simulink model "Drone"  (R2026a)
settings: Solver=VariableStepAuto  StopTime=50
values from neighbouring files (symbols this model uses):
  b = 3.13*10^(-5)    (= 3.13e-05)    [Drone_parameters.m]
  d = 7.5*10^(-7)    (= 7.5e-07)    [Drone_parameters.m]
  g = 9.81    [Drone_parameters.m]
  Ir = 6.5*10^(-5)    (= 6.5e-05)    [Drone_parameters.m]
  Ix = 7.5*10^(-3)    (= 0.0075)    [Drone_parameters.m]
  Iy = 7.5*10^(-3)    (= 0.0075)    [Drone_parameters.m]
  Iz = 1.3*10^(-2)    (= 0.013)    [Drone_parameters.m]
  kx = 0.01    [Drone_parameters.m]
  l = 0.23    [Drone_parameters.m]
  m = 0.65    [Drone_parameters.m]
libraries: slpidlib x6
settings Model: Creator=azmeh  LastModifiedBy=azmeh

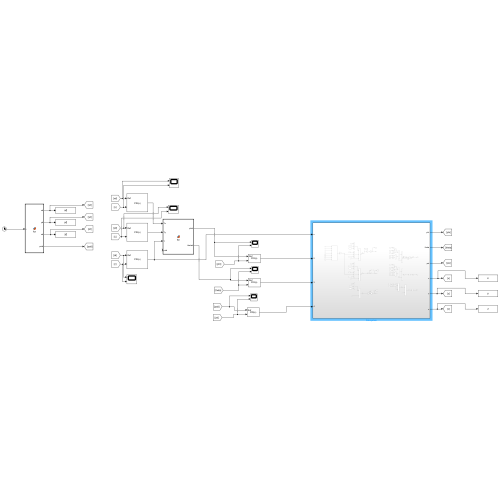
[thumbnail: Simulink's stored preview of the top-level diagram]
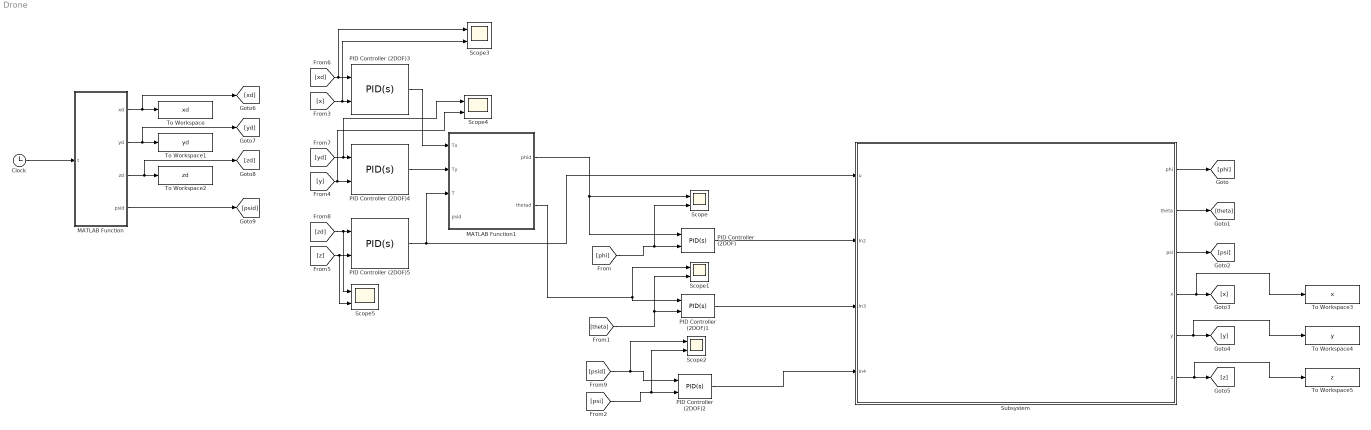
== system Drone ==
  Clock : Clock
  MATLAB Function : MATLAB Function  TreatAsAtomicUnit=on
  MATLAB Function1 : MATLAB Function  TreatAsAtomicUnit=on
  PID Controller (2DOF){,1..5} (6 alike) : slpidlib/PID Controller (2DOF)  Controller=PID  Form=Parallel  TimeDomain=Continuous-time  UseExternalTs=off  SampleTime=-1  IntegratorMethod=Forward Euler  FilterMethod=Forward Euler  ControllerParametersSource=internal  P=5  I=5  UseKiTs=off  D=5  UseExternalDerivativeSource=off  N=100  UseFilter=on  b=1  c=1  TunerSelectOption=Transfer Function Based (PID Tuner App)  InitialConditionSource=internal  InitialConditionForIntegrator=0  InitialConditionForFilter=0  DifferentiatorICPrevScaledInput=0  ExternalReset=none  TrackingMode=off  Kt=1  LimitOutput=off  SatLimitsSource=internal  UpperSaturationLimit=inf  LowerSaturationLimit=-inf  LinearizeAsGain=on  AntiWindupMode=none  Kb=1  LimitIntegrator=off  UpperIntegratorSaturationLimit=inf  LowerIntegratorSaturationLimit=-inf  POutMin=[]  POutMax=[]  IOutMin=[]  IOutMax=[]  DOutMin=[]  DOutMax=[]  NOutMin=[]  NOutMax=[]  bOutMin=[]  bOutMax=[]  cOutMin=[]  cOutMax=[]  SumOutMin=[]  SumOutMax=[]  SaturationOutMin=[]  SaturationOutMax=[]  PParamMin=[]  PParamMax=[]  IParamMin=[]  IParamMax=[]  DParamMin=[]  DParamMax=[]  NParamMin=[]  NParamMax=[]  bParamMin=[]  bParamMax=[]  cParamMin=[]  cParamMax=[]  KbParamMin=[]  KbParamMax=[]  KtParamMin=[]  KtParamMax=[]  KbOutMin=[]  KbOutMax=[]  KtOutMin=[]  KtOutMax=[]  IntegratorOutMin=[]  IntegratorOutMax=[]  FilterOutMin=[]  FilterOutMax=[]  SumI1OutMin=[]  SumI1OutMax=[]  SumI2OutMin=[]  SumI2OutMax=[]  SumI3OutMin=[]  SumI3OutMax=[]  SumI4OutMin=[]  SumI4OutMax=[]  SumDOutMin=[]  SumDOutMax=[]  Sum1OutMin=[]  Sum1OutMax=[]  Sum2OutMin=[]  Sum2OutMax=[]  Sum3OutMin=[]  Sum3OutMax=[]  DifferentiatorOutMin=[]  DifferentiatorOutMax=[]  FilterDiffOutCoefMin=[]  FilterDiffOutCoefMax=[]  ReciprocalOutMin=[]  ReciprocalOutMax=[]  SumDenOutMin=[]  SumDenOutMax=[]  SumNumOutMin=[]  SumNumOutMax=[]  DivideOutMin=[]  DivideOutMax=[]  UdiffTsProdOutMin=[]  UdiffTsProdOutMax=[]  NTsProdOutMin=[]  NTsProdOutMax=[]  UintegralTsProdOutMin=[]  UintegralTsProdOutMax=[]  UngainTsProdOutMin=[]  UngainTsProdOutMax=[]  ClampingZeroOutDataTypeStr=Inherit: Inherit via back propagation  ClampingZeroOutMin=[]  ClampingZeroOutMax=[]  FilterDenConstantOutDataTypeStr=Inherit: Inherit via back propagation  FilterDenConstantOutMin=[]  FilterDenConstantOutMax=[]  PCopyOutDataTypeStr=Inherit: Inherit via back propagation  PCopyOutMin=[]  PCopyOutMax=[]  NCopyOutDataTypeStr=Inherit: Inherit via back propagation  NCopyOutMin=[]  NCopyOutMax=[]  IntegratorContinuousStateAttributes=''  IntegratorStateMustResolveToSignalObject=off  IntegratorRTWStateStorageClass=Auto  FilterContinuousStateAttributes=''  FilterStateMustResolveToSignalObject=off  FilterRTWStateStorageClass=Auto  ParallelPVariant=InternalParameters  IdealPVariant=Disabled  IVariant=InternalParameters  DVariant=InternalParameters  bVariant=InternalParameters  cVariant=InternalParameters  IntegratorVariant=Continuous  SatVariant=Disabled  AWVariant=Passthrough  PCopyVariant=Disabled  TRVariant=Disabled  FdbkBlocksVariant=Forward  IdealPFdbkVariant=Disabled  SatFdbkVariant=Disabled  DerivativeFilterVariant=ContFilter  NVariant=InternalParameters  NCopyVariant=Disabled  FilterICVariant=InternalICsFilter  IntegratorICVariant=InternalICs  ExternalResetVariant=Disabled  TRSumVariant=Passthrough  SumFdbkVariant=Disabled  SumVariant=Sum_PID  TsampFilterVariant=InternalTs  TsampNgainVariant=Passthrough  TsampIntegralVariant=Disabled_SignalSpec  ExternalSaturationOutDataTypeStr=Inherit: Same as second input  DerivativeSourceVariant=ErrorSignal  PreIntVariant=InternalPreInt
  Scope{,1..5} (6 alike) : Scope  NumInputPorts=2
      Scope settings: ActiveDisplayYMinimum=-1.2516778328398153  ActiveDisplayYMaximum=1.2517823015817509
      Scope1 settings: ActiveDisplayYMinimum=-1.2516778328398153  ActiveDisplayYMaximum=1.2517823015817509
      Scope2 settings: ActiveDisplayYMinimum=-1.2516778328398153  ActiveDisplayYMaximum=1.2517823015817509  DataLoggingVariableName=ScopeData2
      Scope3 settings: ActiveDisplayYMinimum=-1.251200752128635  ActiveDisplayYMaximum=1.2513999576485162  DataLoggingVariableName=ScopeData3
      Scope4 settings: ActiveDisplayYMinimum=-1  ActiveDisplayYMaximum=1  DataLoggingVariableName=ScopeData4
      Scope5 settings: ActiveDisplayYMinimum=-1  ActiveDisplayYMaximum=1  DataLoggingVariableName=ScopeData5
  Subsystem : Subsystem
  To Workspace : ToWorkspace  VariableName=xd  SampleTime=-1
  To Workspace1 : ToWorkspace  VariableName=yd  SampleTime=-1
  To Workspace2 : ToWorkspace  VariableName=zd  SampleTime=-1
  To Workspace3 : ToWorkspace  VariableName=x  SampleTime=-1
  To Workspace4 : ToWorkspace  VariableName=y  SampleTime=-1
  To Workspace5 : ToWorkspace  VariableName=z  SampleTime=-1
  wires:
  Subsystem/1(phi) -> [phi]
  MATLAB Function1/1(phid) -> Scope/1, PID Controller (2DOF)/1
  [phi] -> Scope/2, PID Controller (2DOF)/2
  PID Controller (2DOF)/1 -> Subsystem/2(In2)
  Subsystem/2(theta) -> [theta]
  Subsystem/3(psi) -> [psi]
  PID Controller (2DOF)1/1 -> Subsystem/3(In3)
  [theta] -> PID Controller (2DOF)1/2, Scope1/2
  MATLAB Function1/2(thetad) -> PID Controller (2DOF)1/1, Scope1/1
  [psid] -> Scope2/1, PID Controller (2DOF)2/1
  [psi] -> Scope2/2, PID Controller (2DOF)2/2
  PID Controller (2DOF)2/1 -> Subsystem/4(In4)
  Clock/1 -> MATLAB Function/1(t)
  MATLAB Function/1(xd) -> [xd], To Workspace/1
  MATLAB Function/3(zd) -> [zd], To Workspace2/1
  MATLAB Function/2(yd) -> [yd], To Workspace1/1
  Subsystem/4(x) -> To Workspace3/1, [x]
  Subsystem/5(y) -> To Workspace4/1, [y]
  Subsystem/6(z) -> To Workspace5/1, [z]
  [xd] -> Scope3/1, PID Controller (2DOF)3/1
  [x] -> Scope3/2, PID Controller (2DOF)3/2
  [yd] -> Scope4/1, PID Controller (2DOF)4/1
  [y] -> PID Controller (2DOF)4/2, Scope4/2
  [zd] -> Scope5/1, PID Controller (2DOF)5/1
  [z] -> Scope5/2, PID Controller (2DOF)5/2
  MATLAB Function/4(psid) -> [psid]
  PID Controller (2DOF)3/1 -> MATLAB Function1/1(Tx)
  PID Controller (2DOF)4/1 -> MATLAB Function1/2(Ty)
  PID Controller (2DOF)5/1 -> MATLAB Function1/3(T), Subsystem/1(u)

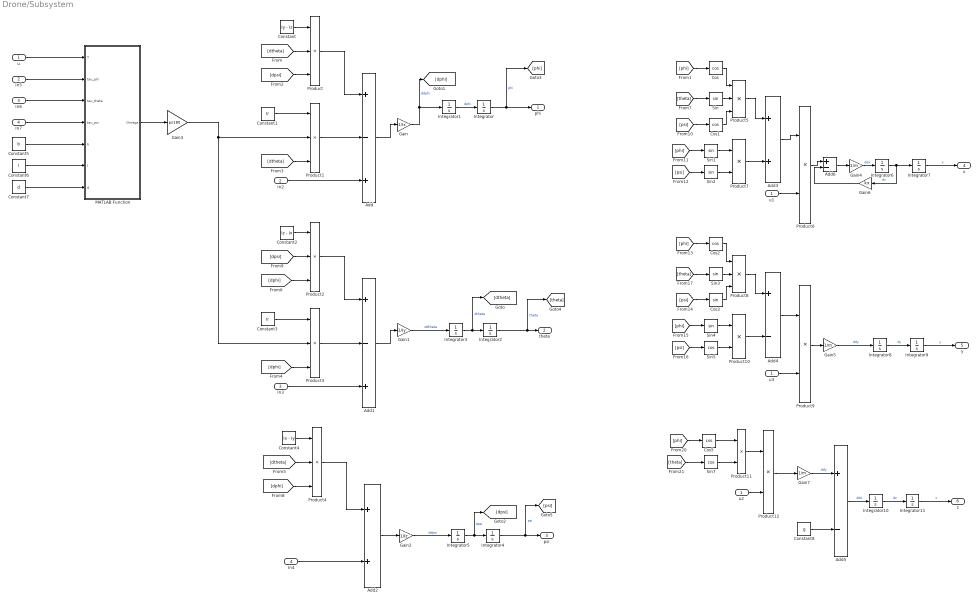
== system Drone/Subsystem ==
  u : Inport
  In2 : Inport  Port=2
  In3 : Inport  Port=3
  In4 : Inport  Port=4
  Add : Sum  Inputs=+-+
  Add1 : Sum  Inputs=+-+
  Add2 : Sum
  Add3 : Sum
  Add4 : Sum  Inputs=+-
  Add5 : Sum  Inputs=+-
  Add6 : Sum  Inputs=+-
  Constant : Constant  Value=Iy - Iz
  Constant1 : Constant  Value=Ir
  Constant2 : Constant  Value=Iz - Ix
  Constant3 : Constant  Value=Ir
  Constant4 : Constant  Value=Ix - Iy
  Constant5 : Constant  Value=b
  Constant6 : Constant  Value=l
  Constant7 : Constant  Value=d
  Constant8 : Constant  Value=g
  Cos{,1..2,5} (4 alike) : Trigonometry  Operator=cos
  Cos3 : Trigonometry
  Gain : Gain  Gain=1/Ix
  Gain1 : Gain  Gain=1/Iy
  Gain2 : Gain  Gain=1/Iz
  Gain3 : Gain  Gain=pi/180
  Gain4 : Gain  Gain=1/m
  Gain5 : Gain  Gain=1/m
  Gain6 : Gain  Gain=kx
  Gain7 : Gain  Gain=1/m
  In5 : InportShadow  Port=2
  In6 : InportShadow  Port=3
  In7 : InportShadow  Port=4
  Integrator{,1..6,8..11} (11 alike) : Integrator
  Integrator7 : Integrator  InitialCondition=1
  MATLAB Function : MATLAB Function  TreatAsAtomicUnit=on
  Product{,1..5,8} (7 alike) : Product  Inputs=3
  Product{6..7,9..12} (6 alike) : Product
  Sin{,1..4} (5 alike) : Trigonometry
  Sin5 : Trigonometry  Operator=cos
  Sin7 : Trigonometry  Operator=cos
  u1 : InportShadow
  u2 : InportShadow
  u3 : InportShadow
  phi : Outport
  theta : Outport  Port=2
  psi : Outport  Port=3
  x : Outport  Port=4
  y : Outport  Port=5
  z : Outport  Port=6
  wires:
  Integrator4/1 -> [psi], psi/1  "psi"
  Add/1 -> Gain/1
  [dpsi] -> Product/3
  Add2/1 -> Gain2/1
  MATLAB Function/1(Omega) -> Gain3/1
  Constant4/1 -> Product4/1
  Gain1/1 -> Integrator3/1  "ddtheta"
  Product3/1 -> Add1/2
  Constant2/1 -> Product2/1
  Constant1/1 -> Product1/1
  Constant/1 -> Product/1
  [dphi] -> Product2/3
  Integrator5/1 -> [dpsi], Integrator4/1  "dpsi"
  Integrator3/1 -> [dtheta], Integrator2/1  "dtheta"
  Integrator1/1 -> Integrator/1  "dphi"
  [dtheta] -> Product1/3
  Gain2/1 -> Integrator5/1  "ddpsi"
  Product4/1 -> Add2/1
  [dphi] -> Product4/3
  [dtheta] -> Product4/2
  [dphi] -> Product3/3
  Product/1 -> Add/1
  Gain/1 -> [dphi], Integrator1/1  "ddphi"
  [dpsi] -> Product2/2
  In2/1 -> Add/3
  [dtheta] -> Product/2
  Product2/1 -> Add1/1
  In4/1 -> Add2/2
  Constant3/1 -> Product3/1
  Add1/1 -> Gain1/1
  Product1/1 -> Add/2
  In3/1 -> Add1/3
  Integrator/1 -> [phi], phi/1  "phi"
  Integrator2/1 -> [theta], theta/1  "theta"
  u/1 -> MATLAB Function/1(T)
  In5/1 -> MATLAB Function/2(tau_phi)
  In6/1 -> MATLAB Function/3(tau_theta)
  In7/1 -> MATLAB Function/4(tau_psi)
  Constant5/1 -> MATLAB Function/5(b)
  Constant6/1 -> MATLAB Function/6(l)
  Constant7/1 -> MATLAB Function/7(d)
  Gain3/1 -> Product3/2, Product1/2
  Integrator6/1 -> Gain6/1, Integrator7/1  "dx"
  Integrator7/1 -> x/1  "x"
  Gain4/1 -> Integrator6/1  "ddx"
  Gain5/1 -> Integrator8/1  "ddy"
  Integrator9/1 -> y/1  "y"
  Integrator8/1 -> Integrator9/1  "dy"
  Integrator10/1 -> Integrator11/1  "dz"
  Integrator11/1 -> z/1  "z"
  Add5/1 -> Integrator10/1  "ddz"
  Add3/1 -> Product6/1
  [phi] -> Cos/1
  [theta] -> Sin/1
  [psi] -> Cos1/1
  Sin/1 -> Product5/2
  Cos/1 -> Product5/1
  Cos1/1 -> Product5/3
  Product5/1 -> Add3/1
  [phi] -> Sin1/1
  [psi] -> Sin2/1
  Sin1/1 -> Product7/1
  Sin2/1 -> Product7/2
  Product7/1 -> Add3/2
  u1/1 -> Product6/2
  u3/1 -> Product9/2
  Product10/1 -> Add4/2
  Sin5/1 -> Product10/2
  Sin4/1 -> Product10/1
  [psi] -> Sin5/1
  [phi] -> Sin4/1
  Product8/1 -> Add4/1
  Cos3/1 -> Product8/3
  Cos2/1 -> Product8/1
  Sin3/1 -> Product8/2
  [psi] -> Cos3/1
  [theta] -> Sin3/1
  [phi] -> Cos2/1
  Add4/1 -> Product9/1
  Product9/1 -> Gain5/1
  Gain7/1 -> Add5/1  "ddy"
  Product12/1 -> Gain7/1
  Constant8/1 -> Add5/2
  Sin7/1 -> Product11/2
  Cos5/1 -> Product11/1
  [theta] -> Sin7/1
  [phi] -> Cos5/1
  Product11/1 -> Product12/1
  u2/1 -> Product12/2
  Add6/1 -> Gain4/1
  Product6/1 -> Add6/1
  Gain6/1 -> Add6/2

== matlab function Drone/MATLAB Function ==
  data: t input; xd output; yd output; zd output; psid output
function [xd, yd, zd, psid] = fcn(t)

xd = cos(0.2*t);
yd = sin(0.2*t);
zd = 10*t;
psid = sin(t);

== matlab function Drone/Subsystem/MATLAB Function ==
  data: T input; Omega output; tau_phi input; tau_theta input; tau_psi input; b input; l input; d input
function Omega = fcn(T, tau_phi, tau_theta, tau_psi, b, l, d)

U1 = T/b;
U2 = tau_phi/l*b;
U3 = tau_theta/l*b;
U4 = tau_psi/d;

omega_3 = sqrt(max(0, (U1 + U4 + 2*U2)/4));
omega_1 = sqrt(max(0, (U1 + U4 - 2*U2)/4));
omega_4 = sqrt(max(0, (U1 - U4 + 2*U3)/4));
omega_2 = sqrt(max(0, (U1 + U4 - 2*U3)/4));

Omega = omega_1 - omega_2 + omega_3 - omega_4;

== matlab function Drone/MATLAB Function1 ==
  data: Tx input; phid output; Ty input; T input; psid input; thetad output
function [phid, thetad] = fcn(Tx, Ty, T, psid)

phid = (Tx*sin(psid) - Ty*cos(psid))/T;
thetad = ((Tx*cos(psid) + Ty*sin(psid))/cos(phid))/T;

phid = max(phid, -pi/6);
phid = min(phid, pi/6);

thetad = max(thetad, -pi/6);
thetad = min(thetad, pi/6);
